simulink model "MBD_Logic_Operations"  (R2021b)
settings: Solver=FixedStepDiscrete  StartTime=0.0  StopTime=10.0  FixedStep=0.001  RelTol=1e-3
libraries: simulink x5
settings Model: Creator=waleed.elshemy  LastModifiedBy=waleed.elshemy
settings OptimizationCC: DefaultParameterBehavior=Inlined  UseDivisionForNetSlopeComputation=on  GainParamInheritBuiltInType=on  UseFloatMulNetSlope=on  InlineInvariantSignals=on  PassReuseOutputArgsAs=Individual arguments  ZeroExternalMemoryAtStartup=off  ZeroInternalMemoryAtStartup=off  NoFixptDivByZeroProtection=on  EfficientFloat2IntCast=on  LifeSpan=1  OptimizeBlockOrder=speed  DifferentSizesBufferReuse=on  EfficientTunableParamExpr=on
settings DebuggingCC: ParameterTunabilityLossMsg=error
settings HardwareCC: ProdLongLongMode=on
settings SFSimCC: MATLABDynamicMemAlloc=off
settings RTWCC: Description=Embedded Coder  SystemTargetFile=ert.tlc  TemplateMakefile=ert_default_tmf
settings CodeAppCC: ForceParamTrailComments=on  IgnoreCustomStorageClasses=off  OperatorAnnotations=on  SimulinkDataObjDesc=on  SFDataObjDesc=on  CustomSymbolStrGlobalVar=rt$N$M  CustomSymbolStrType=$N$M  CustomSymbolStrFcn=$N$M$F  CustomSymbolStrMacro=$N$M  InsertBlockDesc=on
settings ERTTargetCC: TargetLangStandard=C99 (ISO)  GenerateSampleERTMain=on  IncludeMdlTerminateFcn=off  CombineSignalStateStructs=on  SupportComplex=off  SupportContinuousTime=on  InlinedParameterPlacement=NonHierarchical  ERTCustomFileTemplate=example_file_process.tlc  ERTFilePackagingFormat=CompactWithDataFile

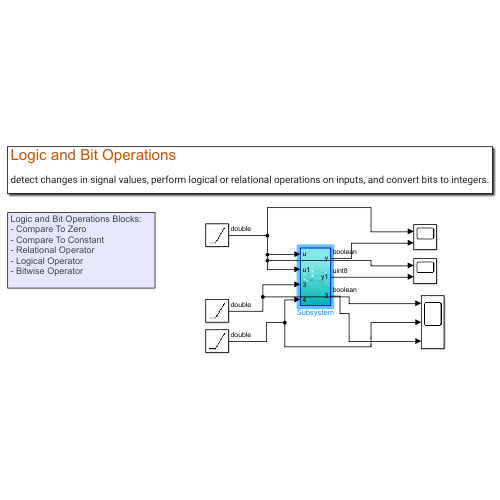
[thumbnail: Simulink's stored preview of the top-level diagram]
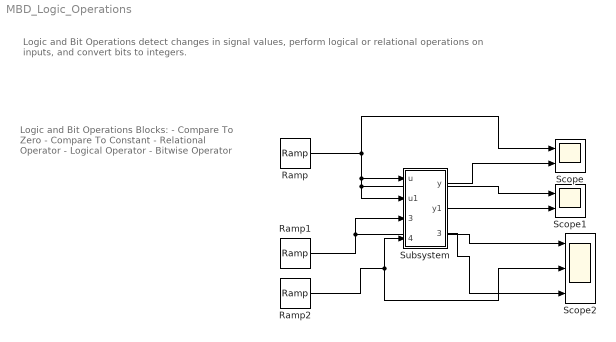
== system MBD_Logic_Operations ==
  note: Logic and Bit Operations
      | detect changes in signal values, perform logical or relational operations on inputs, and convert bits to integers.
  note: Logic and Bit Operations Blocks:
      | - Compare To Zero
      | - Compare To Constant
      | - Relational Operator
      | - Logical Operator
      | - Bitwise Operator
  Ramp : simulink/Sources/Ramp  slope=1  start=0  InitialOutput=-4
  Ramp1 : simulink/Sources/Ramp  slope=1  start=0  InitialOutput=0
  Ramp2 : simulink/Sources/Ramp  slope=-1  start=0  InitialOutput=10
  Scope : Scope  NumInputPorts=2
  Scope1 : Scope  NumInputPorts=2
  Scope2 : Scope  NumInputPorts=3
  Subsystem : Subsystem
  wires:
  Ramp/1 -> Subsystem/1(u), Subsystem/2(u1), Scope1/1, Scope/1
  Ramp2/1 -> Subsystem/4(In4), Scope2/2
  Ramp1/1 -> Subsystem/3(In3), Scope2/1
  Subsystem/1(y) -> Scope/2
  Subsystem/2(y1) -> Scope1/2
  Subsystem/3(Out3) -> Scope2/3

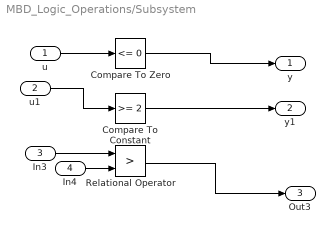
== system MBD_Logic_Operations/Subsystem ==
  u : Inport
  u1 : Inport  Port=2
  In3 : Inport  Port=3
  In4 : Inport  Port=4
  Compare To Constant : simulink/Logic and Bit Operations/Compare To Constant  relop=>=  const=2  OutDataTypeStr=uint8
  Compare To Zero : simulink/Logic and Bit Operations/Compare To Zero  relop=<=  OutDataTypeStr=boolean
  Relational Operator : RelationalOperator  Operator=>  OutDataTypeStr=boolean  RndMeth=Simplest
  y : Outport
  y1 : Outport  Port=2
  Out3 : Outport  Port=3
  wires:
  Compare To Zero/1 -> y/1
  Relational Operator/1 -> Out3/1
  In3/1 -> Relational Operator/1
  u/1 -> Compare To Zero/1
  In4/1 -> Relational Operator/2
  Compare To Constant/1 -> y1/1
  u1/1 -> Compare To Constant/1
